simulink model "issue_2054062_model"  (Simulink 9.2)
settings: Solver=FixedStepDiscrete  StartTime=0.0  StopTime=0.0  FixedStep=1  RelTol=1e-3
InitFcn:
  |    f1 = Simulink.BusElement();
  |    f1.Name = 'f1';
  |    f1.DataType = 'int32';
  |    f2 = f1;
  |    f2.Name = 'f2';
  |    f3 = f2;
  |    f3.Name = 'f3';
  |    f4 = f3;
  |    f4.Name = 'f4';
  | 
  |    struct_T = Simulink.Bus();
  |    struct_T.Elements = [f1,f2,f3,f4];
  |    A = struct(...
  |         'f1',{int32(1),int32(0),int32(0),int32(0)},...
  |         'f2',{int32(0),int32(2),int32(0),int32(0)},...
  |         'f3',{int32(0),int32(0),int32(3),int32(0)},...
  |         'f4',{int32(0),int32(0),int32(0),int32(0)});
settings Model: Creator=ksurende  LastModifiedBy=汪海博
settings DataIOCC: LimitDataPoints=off  SaveFormat=Structure  SignalLoggingSaveFormat=Dataset  ReturnWorkspaceOutputs=on
settings OptimizationCC: RollThreshold=0
settings DebuggingCC: UnderspecifiedInitializationDetection=Simplified  MergeDetectMultiDrivingBlocksExec=error  FcnCallInpInsideContextMsg=error  StateNameClashWarn=none  SFUnexpectedBacktrackingDiag=error  SFNoUnconditionalDefaultTransitionDiag=error
settings HardwareCC: ProdBitPerPointer=64  ProdLargestAtomicFloat=Float  ProdIntDivRoundTo=Zero  ProdEndianess=LittleEndian  ProdLongLongMode=on  ProdHWDeviceType=Specified  TargetBitPerPointer=64  TargetBitPerSizeT=64  TargetBitPerPtrDiffT=64  TargetLongLongMode=on  TargetIntDivRoundTo=Zero  TargetEndianess=LittleEndian  TargetWordSize=64  TargetHWDeviceType=Generic->MATLAB Host Computer  ProdEqTarget=off
settings ModelReferenceCC: PropagateSignalLabelsOutOfModel=on
settings SFSimCC: SimUseLocalCustomCode=on
settings RTWCC: RTWUseLocalCustomCode=on
settings GRTTargetCC: TargetLangStandard=C99 (ISO)  GeneratePreprocessorConditionals=Use local settings  CombineOutputUpdateFcns=on  GRTInterface=off  MultiInstanceErrorCode=None
settings ConfigComp: CovMetricSettings=dwe  CovHtmlReporting=off  CovSaveCumulativeToWorkspaceVar=off  CovSaveSingleToWorkspaceVar=off  CovExternalEMLEnable=on

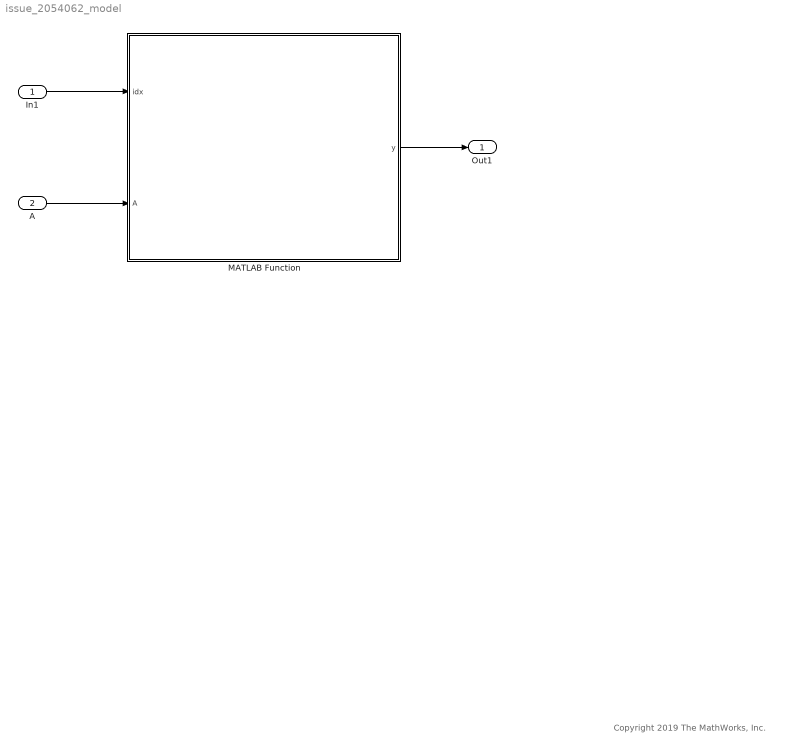
== system issue_2054062_model ==
  note: Copyright 2019 The MathWorks, Inc.
  In1 : Inport  OutDataTypeStr=int32
  A : Inport  Port=2  OutDataTypeStr=Bus:struct_T  PortDimensions=4  BusOutputAsStruct=on
  MATLAB Function : MATLAB Function  TreatAsAtomicUnit=on
  Out1 : Outport
  wires:
  In1/1 -> MATLAB Function/1(idx)
  MATLAB Function/1(y) -> Out1/1
  A/1 -> MATLAB Function/2(A)

== matlab function MATLAB Function ==
  data: idx input double; y output double; A input double
function y = fcn(idx,A)
y = zeros([4,4],'int32');
s1 = A(idx + 1);
y = process(y,s1,A);
end

function y = process(y,s1,A)
coder.inline('never');
for k = 1:4
    if(k == 1)
        s1 = A(s1.f1 + 1);
    elseif(k == 2)
        s1 = A(s1.f2 + 1);
    elseif(k == 3)
        s1 = A(s1.f3 + 1);
    elseif(k == 4)
        s1 = A(s1.f4 + 1);
    end
    y(k,:) = [s1.f1,s1.f2,s1.f3,s1.f4];
end
end
